simulink model "TrajectoryScalingEmulation"  (R2018b)
settings: configuration reference "Active" (kept outside this file)
model workspace (MAT data in the model file):
  Raceline = Simulink.Parameter
  Raceline.DataType = 'auto'
  Raceline.Dimensions = [0 0]
undefined symbols (not defined in the file): EmergencyTrajectory, P_VDC_UseExternalMaxScaleFactor, PerformanceTrajectory, tS
settings Model: DataDictionary=TrajectoryScalingEmulation.sldd  OrderedModelArguments=off  Creator=wischnewski  LastModifiedBy=ge34qer

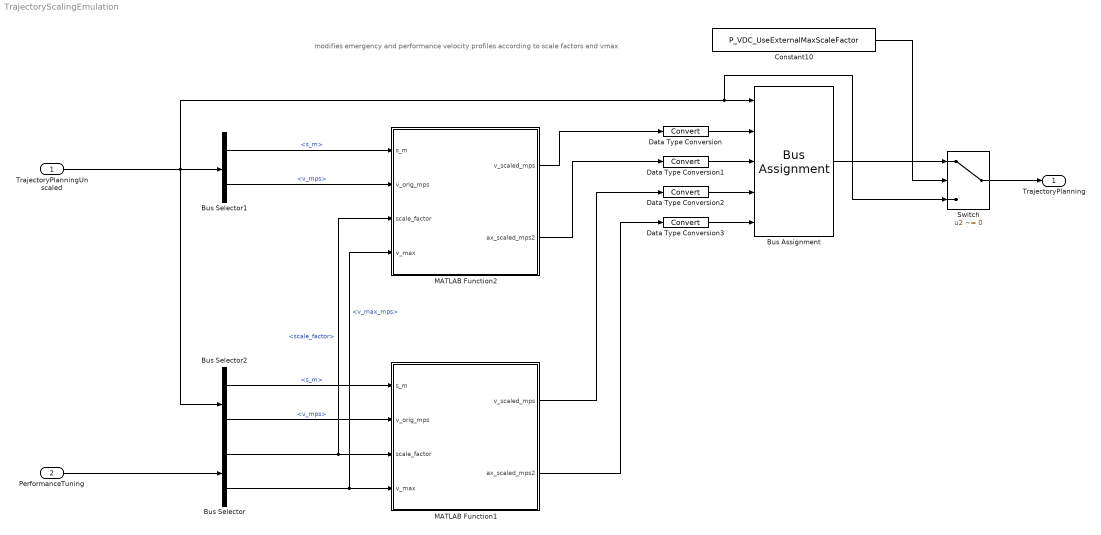
== system TrajectoryScalingEmulation ==
  note: modifies emergency and performance velocity profiles according to scale factors and vmax
  TrajectoryPlanningUnscaled : Inport  OutDataTypeStr=Bus: TrajectoryPlanning  SampleTime=tS
  PerformanceTuning : Inport  Port=2  OutDataTypeStr=Bus: Planning_ControlPerformance_Feedback  SampleTime=tS
  Bus Assignment : BusAssignment  AssignedSignals=EmergencyTrajectory.v_mps,EmergencyTrajectory.ax_mps2,PerformanceTrajectory.v_mps,PerformanceTrajectory.ax_mps2
  Bus Selector : BusSelector  OutputSignals=scale_factor,v_max_mps
  Bus Selector1 : BusSelector  OutputSignals=EmergencyTrajectory.s_m,EmergencyTrajectory.v_mps
  Bus Selector2 : BusSelector  OutputSignals=PerformanceTrajectory.s_m,PerformanceTrajectory.v_mps
  Constant10 : Constant  Value=P_VDC_UseExternalMaxScaleFactor
  Data Type Conversion{,1..3} (4 alike) : DataTypeConversion
  MATLAB Function1 : MATLAB Function  TreatAsAtomicUnit=on
  MATLAB Function2 : MATLAB Function  TreatAsAtomicUnit=on
  Switch : Switch  Criteria=u2 ~= 0
  TrajectoryPlanning : Outport  OutDataTypeStr=Bus: TrajectoryPlanning  SampleTime=tS  BusOutputAsStruct=on
  wires:
  TrajectoryPlanningUnscaled/1 -> Bus Selector2/1, Switch/3, Bus Assignment/1, Bus Selector1/1
  PerformanceTuning/1 -> Bus Selector/1
  Bus Selector/2 -> MATLAB Function2/4(v_max), MATLAB Function1/4(v_max)  "<v_max_mps>"
  Bus Selector/1 -> MATLAB Function1/3(scale_factor), MATLAB Function2/3(scale_factor)  "<scale_factor>"
  Bus Selector1/2 -> MATLAB Function2/2(v_orig_mps)  "<v_mps>"
  Bus Selector1/1 -> MATLAB Function2/1(s_m)  "<s_m>"
  Bus Selector2/1 -> MATLAB Function1/1(s_m)  "<s_m>"
  Bus Selector2/2 -> MATLAB Function1/2(v_orig_mps)  "<v_mps>"
  Data Type Conversion/1 -> Bus Assignment/2
  Data Type Conversion1/1 -> Bus Assignment/3
  Data Type Conversion2/1 -> Bus Assignment/4
  Data Type Conversion3/1 -> Bus Assignment/5
  MATLAB Function2/1(v_scaled_mps) -> Data Type Conversion/1
  MATLAB Function2/2(ax_scaled_mps2) -> Data Type Conversion1/1
  MATLAB Function1/1(v_scaled_mps) -> Data Type Conversion2/1
  MATLAB Function1/2(ax_scaled_mps2) -> Data Type Conversion3/1
  Bus Assignment/1 -> Switch/1
  Constant10/1 -> Switch/2
  Switch/1 -> TrajectoryPlanning/1

== matlab function TrajectoryScalingEmulation/MATLAB Function1 ==
  data: s_m input; v_scaled_mps output; v_orig_mps input; scale_factor input; v_max input; ax_scaled_mps2 output
function [v_scaled_mps, ax_scaled_mps2] = scaleVelocityProfile(s_m, v_orig_mps, scale_factor, v_max)
%#codegen
[v_scaled_mps, ax_scaled_mps2] = scaleVelocityProfile(s_m, v_orig_mps, scale_factor, v_max);

== matlab function TrajectoryScalingEmulation/MATLAB Function2 ==
  data: s_m input; v_scaled_mps output; v_orig_mps input; scale_factor input; v_max input; ax_scaled_mps2 output
function [v_scaled_mps, ax_scaled_mps2] = scaleVelocityProfile(s_m, v_orig_mps, scale_factor, v_max)
%#codegen
[v_scaled_mps, ax_scaled_mps2] = scaleVelocityProfile(s_m, v_orig_mps, scale_factor, v_max);
